simulink model "animationtest"  (R2015b)
settings: Solver=ode45  StartTime=0.0  StopTime=100  RelTol=1e-3
libraries: simulink x3, vrlib x2
settings Model: Creator=rasrack  LastModifiedBy=rasrack

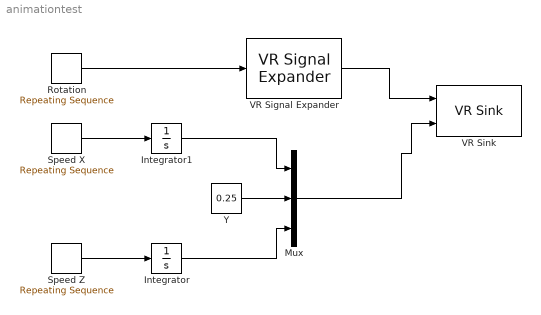
== system animationtest ==
  Integrator : Integrator  UpperSaturationLimit=Inf  LowerSaturationLimit=-Inf  ZeroCross=off
  Integrator1 : Integrator  InitialCondition=3  UpperSaturationLimit=Inf  LowerSaturationLimit=-Inf  ZeroCross=off
  Mux : Mux  Inputs=3
  Rotation : simulink/Sources/Repeating Sequence  rep_seq_t=[0 20 22 80 82 100]  rep_seq_y=[-1.57 -1.57 -0.7 -0.7 0 0]
  Speed X : simulink/Sources/Repeating Sequence  rep_seq_t=[0 20 22 80 82 100]  rep_seq_y=[0 0 0.33 0.33 0.7 0.7]
  Speed Z : simulink/Sources/Repeating Sequence  rep_seq_t=[0 20 22 80 82 100]  rep_seq_y=[0.55 0.55 0.24 0.24 0 0]
  VR Signal Expander : vrlib/VR Signal Expander  outwidth=4  outidx=4
  VR Sink : vrlib/VR Sink  InstantiateOnLoad=on  SampleTime=0.2  ViewEnable=on  RemoteChange=off  RemoteView=off  FieldsWritten=BROV-R_Transform.rotation.4.1.double#BROV-R_Transform.translation.3.1.double  WorldFileName=BROV-R1.wrl  AutoView=off  VideoDimensions=[]  AllowVariableSize=off  FigureProperties="{'Position', 'Name', 'Viewpoint', 'CameraBound', 'CameraDirection', 'CameraPosition', 'CameraUpVector', 'ZoomFactor', 'Antialiasing', 'Headlight', 'Lighting', 'NavPanel', 'Sound', 'StatusBar', 'Stereo3D', 'Stereo3DCameraOffset', 'Stereo3DHIT', 'ToolBar', 'Textures', 'Transparency', 'Triad', 'Wireframe', 'NavZones', 'NavMode', 'NavSpeed', 'CaptureFileFormat', 'CaptureFileName', 'Record2DCompressMethod', 'Record2DCompressQuality', 'Record2D', 'Record2DFileName', 'Record2DFPS'; [1.1000000000000000e+01   1.2000000000000000e+02   5.7600000000000000e+02   3.8000000000000000e+02], '', 'View 1', 'on', [2.8535851488428210e-01   0.0000000000000000e+00   9.5842084596644705e-01], [-6.8045326298003744e+01   0.0000000000000000e+00   2.6745870555184986e+01], [0.0000000000000000e+00   1.0000000000000000e+00   0.0000000000000000e+00], [1.0000000000000000e+00], 'on', 'on', 'on', 'halfbar', 'on', 'on', 'off', [1.0000000149011612e-01], [0.0000000000000000e+00], 'on', 'on', 'on', 'none', 'off', 'off', 'fly', 'normal', 'tif', '%f_anim_%n.tif', 'auto', [7.5000000000000000e+01], 'off', '%f_anim_%n.avi', 'auto'}"
  Y : Constant  Value=0.25
  wires:
  Speed X/1 -> Integrator1/1
  Speed Z/1 -> Integrator/1
  Y/1 -> Mux/2
  Integrator1/1 -> Mux/1
  Integrator/1 -> Mux/3
  Mux/1 -> VR Sink/2
  Rotation/1 -> VR Signal Expander/1
  VR Signal Expander/1 -> VR Sink/1
